simulink model "AUVenv"  (R2025b)
settings: Solver=FixedStepAuto  StartTime=0.0  StopTime=Inf  FixedStep=0.01  RelTol=1e-3
PostLoadFcn:
  | set_param(gcs,'Zoomfactor','fit to view')
undefined symbols (not defined in the file): AUV, fractalcoef, Sim3dSensor, Simple, T200, thrust_pwms, thruster_pose, XYZ
libraries: sim3dlib x7, robotcorelib x5, AUVLib x4, aerolib6dof2 x2, sim3dcameralib x2, matrix_library x1, mspsensorlib x1, aerolibutil x1
(part 1 of 2)
settings Model: Creator=abshanka  LastModifiedBy=ubuntu
settings SolverCC: ZeroCrossAlgorithm=Adaptive
settings DebuggingCC: ReadBeforeWriteMsg=DisableAll  WriteAfterWriteMsg=DisableAll  WriteAfterReadMsg=DisableAll  IgnoredZcDiagnostic=none  MultiTaskDSMMsg=none
settings ModelReferenceCC: UpdateModelReferenceTargets=IfOutOfDate
settings SFSimCC: SFSimEcho=off

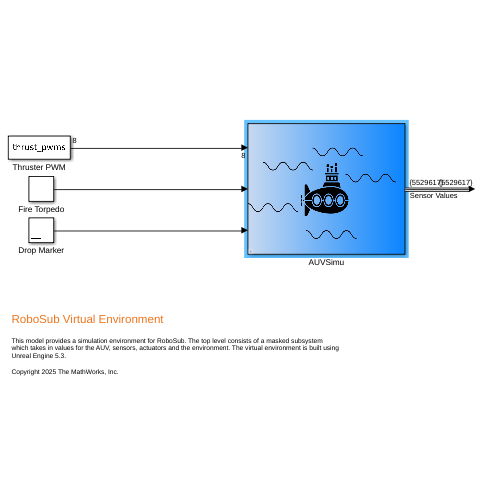
[thumbnail: Simulink's stored preview of the top-level diagram]
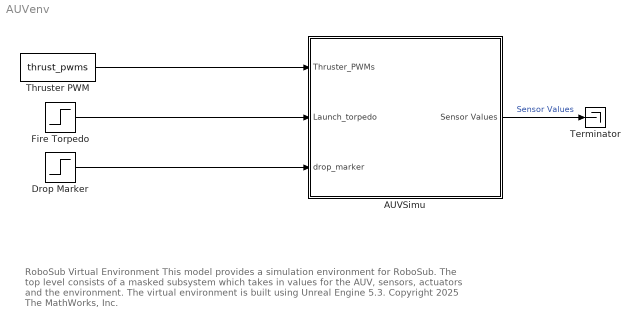
== system AUVenv ==
  note: RoboSub Virtual Environment
      |
      | This model provides a simulation environment for RoboSub. The top level consists of a masked subsystem which takes in values for the AUV, sensors, actuators and the environment. The virtual environment is built using Unreal Engine 5.3.
      |
      | Copyright 2025 The MathWorks, Inc.
  AUVSimu : Subsystem  mask(RoboSub){SourceFile=/home/ubuntu/sonia_control/src/virtual-robosub/fbx files/AUV2.stl, AUV_cob=[0.0026; -0.0004; -0.0911], AUV_height=AUV.Body.hulldiameter, AUV_vol=0.0315, AUV_inertia=AUV.Body.Inertia, AUV_mass=30, AUV_pos=[-142 -142 -1], AUV_orientation=[0 0 pi/2], thruster_pose=thruster_pose, AUV_Voltage=16V, nThrusters=8, Hy=Simple, lin_coeff=diag([ 30,  22,  220]), quad_coeff=diag([ 650,  320,  680]), ang_coeff=diag([ 10, 80,  82]), CMK=AUV.Coeff.CMM, CMM=AUV.Coeff.CMN, CMN=AUV.Coeff.CMK, CZ=AUV.Coeff.CZ, CY=AUV.Coeff.CY, CX=AUV.Coeff.CX, betaR=AUV.IncRange.beta_vec, alphaR=AUV.IncRange.alpha_vec, ang_coeff_c=diag([10, 80, 80]), d_cam_pos=[0 0 -0.26], d_orientation=[0 90 0], SemanticOutportEnabled=off, DepthOutportEnabled=off, TangentialDistortion=[0, 0], RadialDistortion=[0, 0], ImageSize=[720, 1280], OpticalCenter=[640, 360], FocalLength=[1109, 1109], f_cam_pos=[0.5, 0, 0], f_orientation=[0 0 0], SemanticOutportEnabled_f=off, DepthOutportEnabled_f=off, TangentialDistortion_f=[0, 0], RadialDistortion_f=[0, 0], ImageSize_f=[720, 1280], OpticalCenter_f=[640, 360], FocalLength_f=[1109, 1109], ref_mode=Bottom Tracking, Temperature=25, MagneticFieldNED=XYZ, AccelParamsMeasurementRange=Inf, AccelParamsResolution=0, AccelParamsConstantBias=[ 0, 0, 0 ], AccelParamsAxesMisalignment=[ 100, 0, 0; 0, 100, 0; 0, 0, 100 ], AccelParamsNoiseDensity=[ 0, 0, 0 ], AccelParamsBiasInstability=[ 0, 0, 0 ], AccelParamsBiasInstabilityNumerator=fractalcoef().Numerator, AccelParamsBiasInstabilityDenominator=fractalcoef().Denominator, AccelParamsRandomWalk=[ 0, 0, 0 ], AccelParamsNoiseType=double-sided, AccelParamsTemperatureBias=[ 0, 0, 0 ], AccelParamsTemperatureScaleFactor=[ 0, 0, 0 ], GyroParamsMeasurementRange=Inf, GyroParamsResolution=0, GyroParamsConstantBias=[ 0, 0, 0 ], GyroParamsAxesMisalignment=[ 100, 0, 0; 0, 100, 0; 0, 0, 100 ], GyroParamsAccelerationBias=[ 0, 0, 0 ], GyroParamsNoiseDensity=[ 0, 0, 0 ], GyroParamsBiasInstability=[ 0, 0, 0 ], GyroParamsBiasInstabilityNumerator=fractalcoef().Numerator, GyroParamsBiasInstabilityDenominator=fractalcoef().Denominator, GyroParamsRandomWalk=[ 0, 0, 0 ], GyroParamsNoiseType=double-sided, GyroParamsTemperatureBias=[ 0, 0, 0 ], GyroParamsTemperatureScaleFactor=[ 0, 0, 0 ], MagParamsMeasurementRange=Inf, MagParamsResolution=0, MagParamsConstantBias=[ 0, 0, 0 ], MagParamsAxesMisalignment=[ 100, 0, 0; 0, 100, 0; 0, 0, 100 ], MagParamsNoiseDensity=[ 0, 0, 0 ], MagParamsBiasInstability=[ 0, 0, 0 ], MagParamsBiasInstabilityNumerator=fractalcoef().Numerator, MagParamsBiasInstabilityDenominator=fractalcoef().Denominator, MagParamsRandomWalk=[ 0, 0, 0 ], MagParamsNoiseType=double-sided, MagParamsTemperatureBias=[ 0, 0, 0 ], MagParamsTemperatureScaleFactor=[ 0, 0, 0 ], torp_pos=[0.4 0.2 0.1], marker_pos=[-0.01 0 0.02], waterDensity=1000, gravity=9.79624, w_current=None, waterCurrent=[0 0 0], causticsVisibility=off}
      mask prompts: SourceFile "Path to AUV model"; AUV_cob "CoB (relative to CoM) (m)"; AUV_height "Height (or diameter) of AUV (m)"; AUV_vol "Volume of AUV (m^3)"; AUV_inertia "Inerita matrix of AUV"; AUV_mass "Mass of AUV (kg)"; AUV_pos "Inital Position [x,y,z] (m)"; AUV_orientation "Inital Euler Orientation [roll, pith, yaw] (rad)"; thruster_pose "Thruster Pose (nx6 matrix) (m,rad)"; AUV_Voltage "AUV Battery Voltage"; nThrusters "Number of thrusters"; Hy "Choose Hydrodynamics Simulation"; lin_coeff "Linear drag coefficient"; quad_coeff "Quadratic drag coefficient"; ang_coeff "Angular Damping coefficient"; CMK "Rolling moment coeff"; CMM "Pitching moment coeff"; CMN "Yawing moment coeff"; CZ "Normal force coeff (CZ)"; CY "Side force coeff (CY)"; CX "Axial force coeff (CX)"; betaR "Beta Range"; alphaR "Alpha Range"; ang_coeff_c "Angular Damping coefficient"; d_cam_pos "Position (relative to CoM) (m)"; d_orientation "Orientation (deg)"; SemanticOutportEnabled "shared_sim3dblks:sim3dblkCameraPinHole:blkPrm_SemanticOutportEnabled"; DepthOutportEnabled "shared_sim3dblks:sim3dblkCameraPinHole:blkPrm_DepthOutportEnabled"; TangentialDistortion "shared_sim3dblks:sim3dblkCameraPinHole:blkPrm_TangentialDistortion"; RadialDistortion "shared_sim3dblks:sim3dblkCameraPinHole:blkPrm_RadialDistortion"; ImageSize "shared_sim3dblks:sim3dblkCameraPinHole:blkPrm_ImageSize"; OpticalCenter "shared_sim3dblks:sim3dblkCameraPinHole:blkPrm_OpticalCenter"; FocalLength "shared_sim3dblks:sim3dblkCameraPinHole:blkPrm_FocalLength"; f_cam_pos "Position (relative to CoM) (m)"; f_orientation "Orientation (deg)"; SemanticOutportEnabled_f "shared_sim3dblks:sim3dblkCameraPinHole:blkPrm_SemanticOutportEnabled"; DepthOutportEnabled_f "shared_sim3dblks:sim3dblkCameraPinHole:blkPrm_DepthOutportEnabled"; TangentialDistortion_f "shared_sim3dblks:sim3dblkCameraPinHole:blkPrm_TangentialDistortion"; RadialDistortion_f "shared_sim3dblks:sim3dblkCameraPinHole:blkPrm_RadialDistortion"; ImageSize_f "shared_sim3dblks:sim3dblkCameraPinHole:blkPrm_ImageSize"; OpticalCenter_f "shared_sim3dblks:sim3dblkCameraPinHole:blkPrm_OpticalCenter"; FocalLength_f "shared_sim3dblks:sim3dblkCameraPinHole:blkPrm_FocalLength"; ref_mode "Reference mode"; Temperature "Temperature (°C):"; MagneticFieldNED "Magnetic field (NED):"; AccelParamsMeasurementRange "Maximum readings (m/s²):"; AccelParamsResolution "Resolution ((m/s²)/LSB):"; AccelParamsConstantBias "Constant offset bias (m/s²):"; AccelParamsAxesMisalignment "Axes skew (%):"; AccelParamsNoiseDensity "Velocity random walk ((m/s²)/√Hz):"; AccelParamsBiasInstability "Bias instability (m/s²):"; AccelParamsBiasInstabilityNumerator "Bias instability filter numerator coefficients:"; AccelParamsBiasInstabilityDenominator "Bias instability filter denominator coefficients:"; AccelParamsRandomWalk "Acceleration random walk ((m/s²)*√Hz):"; AccelParamsNoiseType "Noise type:"; AccelParamsTemperatureBias "Bias from temperature ((m/s²)/°C):"; AccelParamsTemperatureScaleFactor "Temperature scale factor (%/°C):"; GyroParamsMeasurementRange "Maximum readings (rad/s):"; GyroParamsResolution "Resolution ((rad/s)/LSB):"; GyroParamsConstantBias "Constant offset bias (rad/s):"; GyroParamsAxesMisalignment "Axes skew (%):"; GyroParamsAccelerationBias "Bias from acceleration ((rad/s)/(m/s²)):"; GyroParamsNoiseDensity "Angle random walk ((rad/s)/√Hz):"; GyroParamsBiasInstability "Bias instability (rad/s):"; GyroParamsBiasInstabilityNumerator "Bias instability filter numerator coefficients:"; GyroParamsBiasInstabilityDenominator "Bias instability filter denominator coefficients:"; GyroParamsRandomWalk "Rate random walk ((rad/s)*√Hz):"; GyroParamsNoiseType "Noise type:"; GyroParamsTemperatureBias "Bias from temperature ((rad/s)/°C):"; GyroParamsTemperatureScaleFactor "Temperature scale factor (%/°C):"; MagParamsMeasurementRange "Maximum readings (µT):"; MagParamsResolution "Resolution ((µT)/LSB):"; MagParamsConstantBias "Constant offset bias (µT):"; MagParamsAxesMisalignment "Axes skew (%):"; MagParamsNoiseDensity "White Noise PSD ((µT)/√Hz):"; MagParamsBiasInstability "Bias instability (µT):"; MagParamsBiasInstabilityNumerator "Bias instability filter numerator coefficients:"; MagParamsBiasInstabilityDenominator "Bias instability filter denominator coefficients:"; MagParamsRandomWalk "Random walk ((µT)*√Hz):"; MagParamsNoiseType "Noise type:"; MagParamsTemperatureBias "Bias from temperature ((µT)/°C):"; MagParamsTemperatureScaleFactor "Temperature scale factor (%/°C):"; torp_pos "Torpedo position (m)"; marker_pos "marker_pos (m)"; waterDensity "Water Density (kg/m^3)"; gravity "Acceleration due to Gravity (m/sec^2)"; w_current "Water current"; waterCurrent "Enter current speed in x and y (z=0) (m/s)"; causticsVisibility "Enable Water Caustics"
      mask help:
      | The mask takes in necessary information required to simulate the AUV in a pool. It is divided into 4 sections - AUV Parameters, Sensors, Actuators and Environment.
      | The AUV Parameters section contains all the data related to the AUV body such as mass, inertia, volume, etc. It also takes in the hydrodynamic coefficients (based on the chosen complexity).
      | The Sensors section takes in data related to the sensors such as mounting location and any sensor parameters (for ex: camera - focal lenght, resolution, distortions, etc.)
      | The Actuators sections takes in the mounting location for 2 actuators present in the simulator - torpedo and marker.
      | The Environment section has some parameters related of the environment such as water density, gravity and water currents.
      mask TypeOptions SourceFile: Visualization/AUV mesh/SourceFile
      mask TypeOptions Hy: AUV Dynamics/Environmental Forces and Moments/Hy
      mask TypeOptions lin_coeff: AUV Dynamics/Environmental Forces and Moments/lin_coeff
      mask TypeOptions quad_coeff: AUV Dynamics/Environmental Forces and Moments/quad_coeff
      mask TypeOptions ang_coeff: AUV Dynamics/Environmental Forces and Moments/ang_coeff
      mask TypeOptions CMK: AUV Dynamics/Environmental Forces and Moments/CMK
      mask TypeOptions CMM: AUV Dynamics/Environmental Forces and Moments/CMM
      mask TypeOptions CMN: AUV Dynamics/Environmental Forces and Moments/CMN
      mask TypeOptions CZ: AUV Dynamics/Environmental Forces and Moments/CZ
      mask TypeOptions CY: AUV Dynamics/Environmental Forces and Moments/CY
      mask TypeOptions CX: AUV Dynamics/Environmental Forces and Moments/CX
      mask TypeOptions betaR: AUV Dynamics/Environmental Forces and Moments/betaR
      mask TypeOptions alphaR: AUV Dynamics/Environmental Forces and Moments/alphaR
      mask TypeOptions ang_coeff_c: AUV Dynamics/Environmental Forces and Moments/ang_coeff_c
      mask TypeOptions SemanticOutportEnabled: Sensors/downward_camera/SemanticOutportEnabled
      mask TypeOptions DepthOutportEnabled: Sensors/downward_camera/DepthOutportEnabled
      mask TypeOptions TangentialDistortion: Sensors/downward_camera/TangentialDistortion
      mask TypeOptions RadialDistortion: Sensors/downward_camera/RadialDistortion
      mask TypeOptions ImageSize: Sensors/downward_camera/ImageSize
      mask TypeOptions OpticalCenter: Sensors/downward_camera/OpticalCenter
      mask TypeOptions FocalLength: Sensors/downward_camera/FocalLength
      mask TypeOptions SemanticOutportEnabled_f: Sensors/forward_camera/SemanticOutportEnabled
      mask TypeOptions DepthOutportEnabled_f: Sensors/forward_camera/DepthOutportEnabled
      mask TypeOptions TangentialDistortion_f: Sensors/forward_camera/TangentialDistortion
      mask TypeOptions RadialDistortion_f: Sensors/forward_camera/RadialDistortion
      mask TypeOptions ImageSize_f: Sensors/forward_camera/ImageSize
      mask TypeOptions OpticalCenter_f: Sensors/forward_camera/OpticalCenter
      mask TypeOptions FocalLength_f: Sensors/forward_camera/FocalLength
      mask TypeOptions Temperature: Sensors/IMU Subsystem/IMU/Temperature
      mask TypeOptions MagneticFieldNED: Sensors/IMU Subsystem/IMU/MagneticFieldNED
      mask TypeOptions AccelParamsMeasurementRange: Sensors/IMU Subsystem/IMU/AccelParamsMeasurementRange
      mask TypeOptions AccelParamsResolution: Sensors/IMU Subsystem/IMU/AccelParamsResolution
      mask TypeOptions AccelParamsConstantBias: Sensors/IMU Subsystem/IMU/AccelParamsConstantBias
      mask TypeOptions AccelParamsAxesMisalignment: Sensors/IMU Subsystem/IMU/AccelParamsAxesMisalignment
      mask TypeOptions AccelParamsNoiseDensity: Sensors/IMU Subsystem/IMU/AccelParamsNoiseDensity
      mask TypeOptions AccelParamsBiasInstability: Sensors/IMU Subsystem/IMU/AccelParamsBiasInstability
      mask TypeOptions AccelParamsBiasInstabilityNumerator: Sensors/IMU Subsystem/IMU/AccelParamsBiasInstabilityNumerator
      mask TypeOptions AccelParamsBiasInstabilityDenominator: Sensors/IMU Subsystem/IMU/AccelParamsBiasInstabilityDenominator
      mask TypeOptions AccelParamsRandomWalk: Sensors/IMU Subsystem/IMU/AccelParamsRandomWalk
      mask TypeOptions AccelParamsNoiseType: Sensors/IMU Subsystem/IMU/AccelParamsNoiseType
      mask TypeOptions AccelParamsTemperatureBias: Sensors/IMU Subsystem/IMU/AccelParamsTemperatureBias
      mask TypeOptions AccelParamsTemperatureScaleFactor: Sensors/IMU Subsystem/IMU/AccelParamsTemperatureScaleFactor
      mask TypeOptions GyroParamsMeasurementRange: Sensors/IMU Subsystem/IMU/GyroParamsMeasurementRange
      mask TypeOptions GyroParamsResolution: Sensors/IMU Subsystem/IMU/GyroParamsResolution
      mask TypeOptions GyroParamsConstantBias: Sensors/IMU Subsystem/IMU/GyroParamsConstantBias
      mask TypeOptions GyroParamsAxesMisalignment: Sensors/IMU Subsystem/IMU/GyroParamsAxesMisalignment
      mask TypeOptions GyroParamsAccelerationBias: Sensors/IMU Subsystem/IMU/GyroParamsAccelerationBias
      mask TypeOptions GyroParamsNoiseDensity: Sensors/IMU Subsystem/IMU/GyroParamsNoiseDensity
      mask TypeOptions GyroParamsBiasInstability: Sensors/IMU Subsystem/IMU/GyroParamsBiasInstability
      mask TypeOptions GyroParamsBiasInstabilityNumerator: Sensors/IMU Subsystem/IMU/GyroParamsBiasInstabilityNumerator
      mask TypeOptions GyroParamsBiasInstabilityDenominator: Sensors/IMU Subsystem/IMU/GyroParamsBiasInstabilityDenominator
      mask TypeOptions GyroParamsRandomWalk: Sensors/IMU Subsystem/IMU/GyroParamsRandomWalk
      mask TypeOptions GyroParamsNoiseType: Sensors/IMU Subsystem/IMU/GyroParamsNoiseType
      mask TypeOptions GyroParamsTemperatureBias: Sensors/IMU Subsystem/IMU/GyroParamsTemperatureBias
      mask TypeOptions GyroParamsTemperatureScaleFactor: Sensors/IMU Subsystem/IMU/GyroParamsTemperatureScaleFactor
      mask TypeOptions MagParamsMeasurementRange: Sensors/IMU Subsystem/IMU/MagParamsMeasurementRange
      mask TypeOptions MagParamsResolution: Sensors/IMU Subsystem/IMU/MagParamsResolution
      mask TypeOptions MagParamsConstantBias: Sensors/IMU Subsystem/IMU/MagParamsConstantBias
      mask TypeOptions MagParamsAxesMisalignment: Sensors/IMU Subsystem/IMU/MagParamsAxesMisalignment
      mask TypeOptions MagParamsNoiseDensity: Sensors/IMU Subsystem/IMU/MagParamsNoiseDensity
      mask TypeOptions MagParamsBiasInstability: Sensors/IMU Subsystem/IMU/MagParamsBiasInstability
      mask TypeOptions MagParamsBiasInstabilityNumerator: Sensors/IMU Subsystem/IMU/MagParamsBiasInstabilityNumerator
      mask TypeOptions MagParamsBiasInstabilityDenominator: Sensors/IMU Subsystem/IMU/MagParamsBiasInstabilityDenominator
      mask TypeOptions MagParamsRandomWalk: Sensors/IMU Subsystem/IMU/MagParamsRandomWalk
      mask TypeOptions MagParamsNoiseType: Sensors/IMU Subsystem/IMU/MagParamsNoiseType
      mask TypeOptions MagParamsTemperatureBias: Sensors/IMU Subsystem/IMU/MagParamsTemperatureBias
      mask TypeOptions MagParamsTemperatureScaleFactor: Sensors/IMU Subsystem/IMU/MagParamsTemperatureScaleFactor
      mask DialogControl Container3 Prompt: AUV Parameters
      mask DialogControl Container4 Prompt: General
      mask DialogControl Container5 Prompt: Hydrodynamics
      mask DialogControl Container6 Prompt: Simple hydrodynamics coefficients
      mask DialogControl Container7 Prompt: Complex hydrodynamics coefficients
      mask DialogControl Container8 Prompt: Sensors
      mask DialogControl Container10 Prompt: Downward Camera
      mask DialogControl SemanticOutportEnabled Prompt: Output semantic segmentation
      mask DialogControl DepthOutportEnabled Prompt: Output depth
      mask DialogControl TangentialDistortion Prompt: Tangential distortion coefficients:
      mask DialogControl RadialDistortion Prompt: Radial distortion coefficients:
      mask DialogControl ImageSize Prompt: Image size (pixels):
      mask DialogControl OpticalCenter Prompt: Optical center (pixels):
      mask DialogControl FocalLength Prompt: Focal length (pixels):
      mask DialogControl Container9 Prompt: Forward Camera
      mask DialogControl SemanticOutportEnabled_f Prompt: Output semantic segmentation
      mask DialogControl DepthOutportEnabled_f Prompt: Output depth
      mask DialogControl TangentialDistortion_f Prompt: Tangential distortion coefficients:
      mask DialogControl RadialDistortion_f Prompt: Radial distortion coefficients:
      mask DialogControl ImageSize_f Prompt: Image size (pixels):
      mask DialogControl OpticalCenter_f Prompt: Optical center (pixels):
      mask DialogControl FocalLength_f Prompt: Focal length (pixels):
      mask DialogControl Container11 Prompt: DVL
      mask DialogControl Container12 Prompt: IMU
      mask DialogControl Container16 Prompt: Accelerometer
      mask DialogControl Container17 Prompt: Gyroscope
      mask DialogControl Container18 Prompt: Magnetometer
      mask DialogControl Container13 Prompt: Actuators
      mask DialogControl Container14 Prompt: Environment
      mask Display: image('submarine.png');
  Drop Marker : Step  SampleTime=0
  Fire Torpedo : Step  SampleTime=0
  Terminator : Terminator
  Thruster PWM : Constant  Value=thrust_pwms  SampleTime=0.1
  wires:
  Fire Torpedo/1 -> AUVSimu/2(Launch_torpedo)
  Thruster PWM/1 -> AUVSimu/1(Thruster_PWMs)
  Drop Marker/1 -> AUVSimu/3(drop_marker)
  AUVSimu/1(Sensor Values) -> Terminator/1  "Sensor Values"

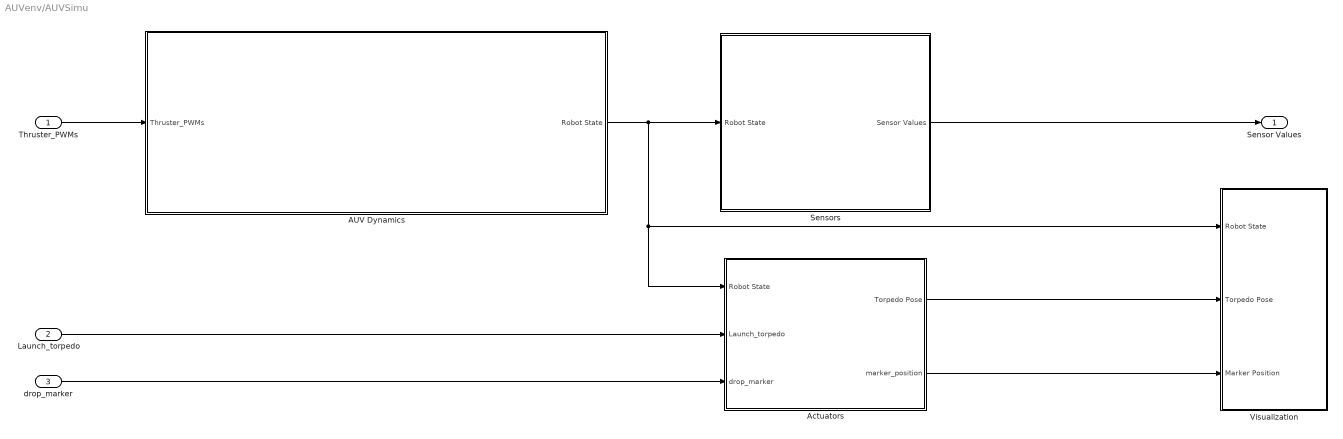
== system AUVenv/AUVSimu ==
  Thruster_PWMs : Inport
  Launch_torpedo : Inport  Port=2
  drop_marker : Inport  Port=3
  AUV Dynamics : Subsystem
  Actuators : Subsystem
  Sensors : Subsystem
  Visualization : Subsystem
  Sensor Values : Outport
  wires:
  Thruster_PWMs/1 -> AUV Dynamics/1(Thruster_PWMs)
  Sensors/1(Sensor Values) -> Sensor Values/1
  AUV Dynamics/1(Robot State) -> Sensors/1(Robot State), Actuators/1(Robot State), Visualization/1(Robot State)
  Launch_torpedo/1 -> Actuators/2(Launch_torpedo)
  drop_marker/1 -> Actuators/3(drop_marker)
  Actuators/1(Torpedo Pose) -> Visualization/2(Torpedo Pose)
  Actuators/2(marker_position) -> Visualization/3(Marker Position)

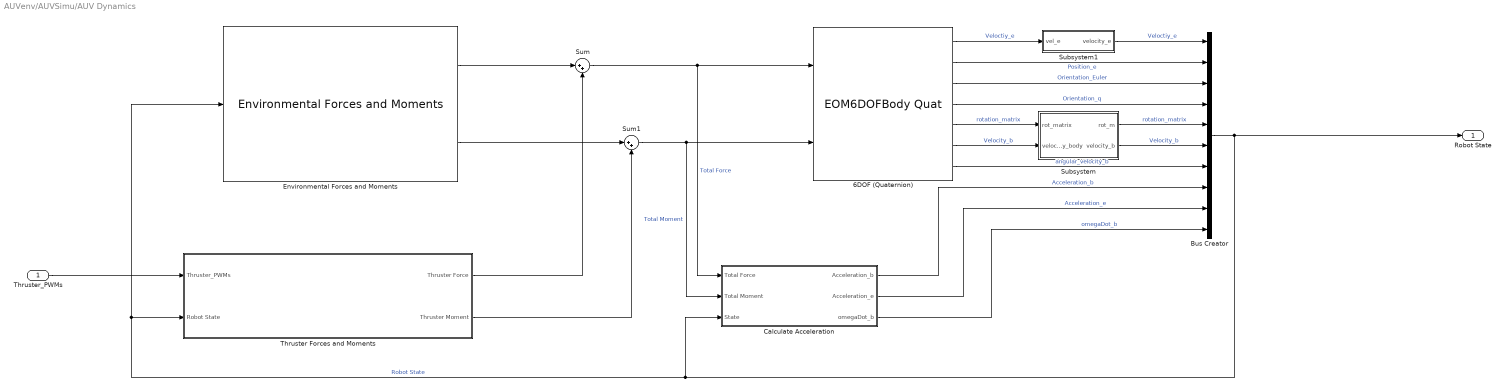
== system AUVenv/AUVSimu/AUV Dynamics ==
  Thruster_PWMs : Inport
  6DOF (Quaternion) : EOM6DOFBodyQuat  xme_0=AUV_pos  eul_0=AUV_orientation  mass_0=AUV_mass  inertia=AUV_inertia
  Bus Creator : BusCreator  Inputs=10
  Calculate Acceleration : Subsystem
  Environmental Forces and Moments : AUVLib/Environmental Forces and Moments  V=AUV_vol  h=AUV_height  mass=AUV_mass  CoB=AUV_cob  Hy=Simple  ang_coeff=ang_coeff  quad_coeff=quad_coeff  lin_coeff=lin_coeff  ang_coeff_c=ang_coeff_c  alphaR=alphaR  betaR=betaR  CX=CX  CY=CY  CZ=CZ  CMK=CMK  CMM=CMM  CMN=CMN  inputAxes=Body  cbar=1  b=1  S=1
  Subsystem : Subsystem
  Subsystem1 : Subsystem
  Sum : Sum  Inputs=|++
  Sum1 : Sum  Inputs=|++
  Thruster Forces and Moments : Subsystem
  Robot State : Outport
  wires:
  6DOF (Quaternion)/3 -> Bus Creator/3  "Orientation_Euler"
  Thruster Forces and Moments/1(Thruster Force) -> Sum/2
  Sum1/1 -> 6DOF (Quaternion)/2, Calculate Acceleration/2(Total Moment)  "Total Moment"
  Thruster Forces and Moments/2(Thruster Moment) -> Sum1/2
  Calculate Acceleration/3(omegaDot_b) -> Bus Creator/10  "omegaDot_b"
  6DOF (Quaternion)/7 -> Bus Creator/7  "angular_velocity_b"
  Sum/1 -> 6DOF (Quaternion)/1, Calculate Acceleration/1(Total Force)  "Total Force"
  Calculate Acceleration/2(Acceleration_e) -> Bus Creator/9  "Acceleration_e"
  6DOF (Quaternion)/1 -> Subsystem1/1(vel_e)  "Veloctiy_e"
  Thruster_PWMs/1 -> Thruster Forces and Moments/1(Thruster_PWMs)
  Calculate Acceleration/1(Acceleration_b) -> Bus Creator/8  "Acceleration_b"
  6DOF (Quaternion)/4 -> Bus Creator/4  "Orientation_q"
  Bus Creator/1 -> Robot State/1, Calculate Acceleration/3(State), Thruster Forces and Moments/2(Robot State), Environmental Forces and Moments/1  "Robot State"
  6DOF (Quaternion)/2 -> Bus Creator/2  "Position_e"
  6DOF (Quaternion)/5 -> Subsystem/1(rot_matrix)  "rotation_matrix"
  6DOF (Quaternion)/6 -> Subsystem/2(velocity_body)  "Velocity_b"
  Subsystem/2(velocity_b) -> Bus Creator/6  "Velocity_b"
  Subsystem/1(rot_m) -> Bus Creator/5  "rotation_matrix"
  Subsystem1/1(velocity_e) -> Bus Creator/1  "Veloctiy_e"
  Environmental Forces and Moments/2 -> Sum1/1
  Environmental Forces and Moments/1 -> Sum/1

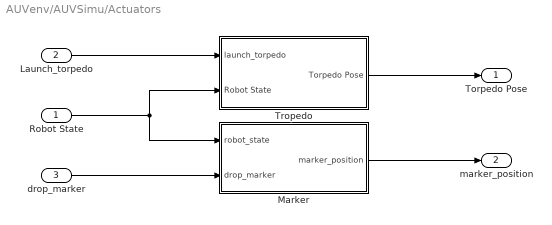
== system AUVenv/AUVSimu/Actuators ==
  Robot State : Inport
  Launch_torpedo : Inport  Port=2
  drop_marker : Inport  Port=3
  Marker : Subsystem
  Tropedo : Subsystem
  Torpedo Pose : Outport
  marker_position : Outport  Port=2
  wires:
  Launch_torpedo/1 -> Tropedo/1(launch_torpedo)
  drop_marker/1 -> Marker/2(drop_marker)
  Robot State/1 -> Marker/1(robot_state), Tropedo/2(Robot State)
  Tropedo/1(Torpedo Pose) -> Torpedo Pose/1
  Marker/1(marker_position) -> marker_position/1

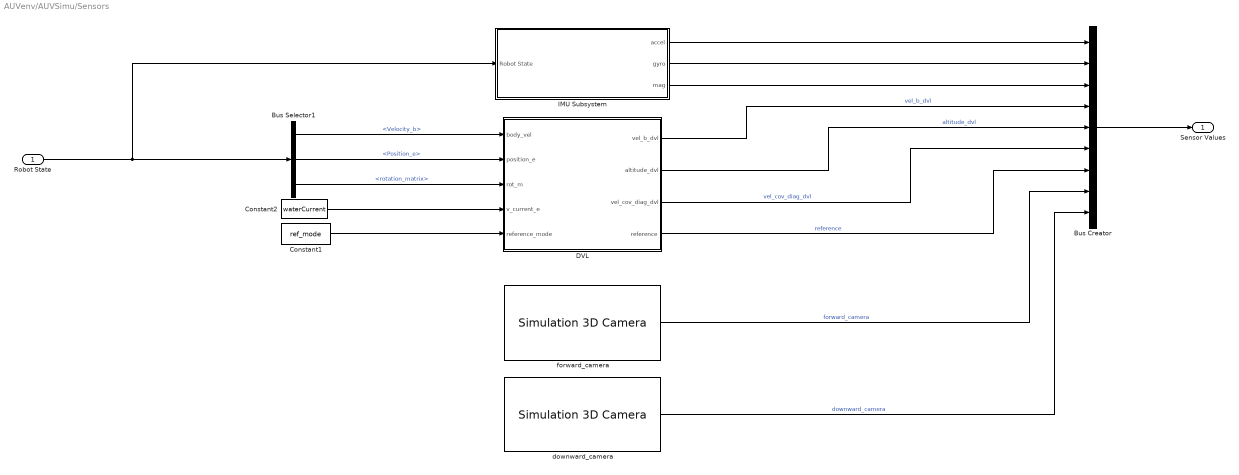
== system AUVenv/AUVSimu/Sensors ==
  Robot State : Inport
  Bus Creator : BusCreator  Inputs=9
  Bus Selector1 : BusSelector  OutputSignals=Velocity_b,Position_e,rotation_matrix
  Constant1 : Constant  Value=ref_mode  OutDataTypeStr=uint8
  Constant2 : Constant  Value=waterCurrent
  DVL : MATLAB Function  TreatAsAtomicUnit=on
  IMU Subsystem : Subsystem
  downward_camera : sim3dcameralib/Simulation 3D Camera  Priority=1  sensorTag=Sim3dSensor�  sensorId=2  sensorName=Sim3dSensor�  vehTagList={'AUVframe';'AUVmesh';'Scene Origin';'marker';'torpedo'}  vehTag=AUVmesh  CoordinateSystem=ISO8855  mountLoc=Origin  offsetFlag=on  tmountOffset=d_cam_pos  extTmount=off  rmountOffset=d_orientation  extRmount=off  FocalLength=FocalLength  OpticalCenter=OpticalCenter  ImageSize=ImageSize  RadialDistortion=RadialDistortion  TangentialDistortion=TangentialDistortion  SensorSkew=0  VisualizeFieldOfView=off  FieldOfViewRange=61  DepthOutportEnabled=off  SemanticOutportEnabled=off  TransformOutportEnabled=off  SampleTime=-1  mountPoint=[0 0 -0.26]  mountOrientation=[0 90 0]  aMode=3  ID=2
      settings: LibrarySourceBlock=drivingsim3d/Simulation 3D Camera
  forward_camera : sim3dcameralib/Simulation 3D Camera  Priority=1  sensorTag=Sim3dSensor�  sensorId=1  sensorName=Sim3dSensor�  vehTagList={'AUVframe';'AUVmesh';'Scene Origin';'marker';'torpedo'}  vehTag=AUVmesh  CoordinateSystem=ISO8855  mountLoc=Origin  offsetFlag=on  tmountOffset=f_cam_pos  extTmount=off  rmountOffset=f_orientation  extRmount=off  FocalLength=FocalLength_f  OpticalCenter=OpticalCenter_f  ImageSize=ImageSize_f  RadialDistortion=RadialDistortion_f  TangentialDistortion=TangentialDistortion_f  SensorSkew=0  VisualizeFieldOfView=off  FieldOfViewRange=61  DepthOutportEnabled=off  SemanticOutportEnabled=off  TransformOutportEnabled=off  SampleTime=-1  mountPoint=[0.5 0 0]  mountOrientation=[0 0 0]  aMode=6  ID=1
      settings: LibrarySourceBlock=robotsim3dlib/Simulation 3D Camera
  Sensor Values : Outport
  wires:
  Robot State/1 -> IMU Subsystem/1(Robot State), Bus Selector1/1
  Bus Selector1/1 -> DVL/1(body_vel)  "<Velocity_b>"
  Bus Selector1/2 -> DVL/2(position_e)  "<Position_e>"
  Bus Selector1/3 -> DVL/3(rot_m)  "<rotation_matrix>"
  Constant2/1 -> DVL/4(v_current_e)
  Constant1/1 -> DVL/5(reference_mode)
  DVL/1(vel_b_dvl) -> Bus Creator/4  "vel_b_dvl"
  DVL/2(altitude_dvl) -> Bus Creator/5  "altitude_dvl"
  DVL/3(vel_cov_diag_dvl) -> Bus Creator/6  "vel_cov_diag_dvl"
  DVL/4(reference) -> Bus Creator/7  "reference"
  Bus Creator/1 -> Sensor Values/1
  forward_camera/1 -> Bus Creator/8  "forward_camera"
  downward_camera/1 -> Bus Creator/9  "downward_camera"
  IMU Subsystem/1(accel) -> Bus Creator/1
  IMU Subsystem/2(gyro) -> Bus Creator/2
  IMU Subsystem/3(mag) -> Bus Creator/3

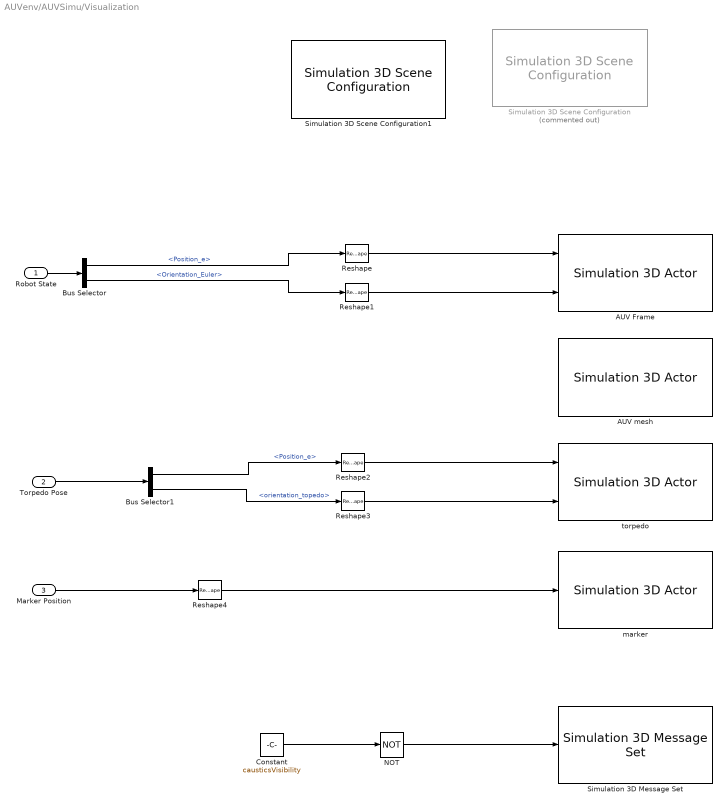
== system AUVenv/AUVSimu/Visualization ==
  Robot State : Inport
  Torpedo Pose : Inport  Port=2
  Marker Position : Inport  Port=3
  AUV Frame : sim3dlib/Simulation 3D Actor  Priority=1  ActorName=AUVframe  ParentName=Scene Origin  Operation=Create at setup  InitScriptText=|  SampleTime=-1  Translation=[0 0 0]  Rotation=[0 0 0]  Scale=[1 1 1]  InputsText=AUVframe.Translation AUVframe.Rotation  aMode=5  ActorTag=AUVframe  ActorType=Sim3dActor  ID=C
      | Actor.CoordinateSystem = 'AERO';
      | Actor.Collisions = false;
  AUV mesh : sim3dlib/Simulation 3D Actor  Priority=1  ActorName=AUVmesh  ParentName=AUVframe  Operation=Create at setup  InitScriptText=|  SampleTime=-1  Translation=[0 0 0]  Rotation=[0 0 0]  Scale=[1 1 1]  aMode=5  ActorTag=AUVmesh  ActorType=Sim3dActor  ID=C
      | Actor.CoordinateSystem = 'AERO';
      | % createShape(Actor, 'Cylinder', [1 0.5 0.5]);
      | Actor.Collisions = false;
  Bus Selector : BusSelector  OutputSignals=Position_e,Orientation_Euler
  Bus Selector1 : BusSelector  OutputSignals=Position_e,orientation_topedo
  Constant : Constant  Value=causticsVisibility  OutDataTypeStr=boolean
  NOT : Logic  Operator=NOT  IconShape=distinctive  AllPortsSameDT=off  OutDataTypeStr=boolean
  Reshape{,1..4} (5 alike) : Reshape  OutputDimensionality=Row vector (2-D)
  Simulation 3D Message Set : sim3dlib/Simulation 3D Message Set  Priority=-1  SigName=causticsVis  Ts=0.01  aMode=0
      settings: LibrarySourceBlock=aerolibsim3d/Simulation 3D Message Set
  Simulation 3D Scene Configuration : sim3dlib/Simulation 3D Scene Configuration  Priority=0  Commented=on  ProjectFormat=Unreal Executable  SceneDesc=Empty scene  ProjectName=/home/ubuntu/simu-sonia/RoboSub_pool_25b/AutoVrtlEnv.exe  ScenePath=/Game/Maps/RoboSub_pool  EnableOpenDRIVE=off  vehTagList={'AUVframe';'AUVmesh';'Custom';'Custom_pool';'Scene Origin';'marker';'torpedo'}  vehTag=Custom_pool  AttachedCameraRelativeTranslation=[0 0 0]  FreeCameraDefaultInitialTranslation=[-6, 0, 2]  AttachedCameraRelativeRotation=[0 0 0]  FreeCameraDefaultInitialRotation=[0, -15, 0]  ViewpointName=Custom_pool  FreeCameraInitialTranslation=[-150 -142 2.5]  ViewpointTranslation=[0 0 0]  FreeCameraInitialRotation=[0 0 0]  ViewpointRotation=[0 0 0]  OpVisEn=off  Ts=.01  EnableWindow=on  EnableRemoteAccess=off  EnableWeather=off  SunAzimuth=90  SunAltitude=40.0  EnableGeospatialSun=off  Latitude=0  Longitude=0  Date=2023-01-01  Time=10:30:00  GeoTimeZone=-5.0  SunDaylightSaving=off  wind=1  clouds=10  EnableVolumetricClouds=off  CloudCoverage=0  CloudAltitude=6  fog=0  rain=0  RaindropsEffect=off  SnowDensity=0  EnableGeospatial=off  TilesetSource=Earth terrain  UseTrueOrigin=off  OriginHeight=200  OriginLatitude=40.744652  OriginLongitude=-73.988864  MapStyle=Aerial  AdditionalAssetIDs=[]  UseAdvancedSunSky=off  SolarTime=11  TimeZone=-5  Day=21  Month=9  Year=2022  UseDaylightSavingTime=on  DSTStartDay=10  DSTStartMonth=3  DSTEndDay=3  DSTEndMonth=11  DSTSwitchHour=2  sensorTag=MainCamera1  sensorId=1  sensorName=MainCamera1  mountLoc=Origin  offsetFlag=off  tmountOffset=[0, 0, 0]  rmountOffset=[0, 0, 0]  HorizontalResolution=1280  VerticalResolution=720  HorizontalFOV=60  mountPoint=[0 0 0]  mountOrientation=[0 0 0]  aMode=5  ID=1  GeoTrigger=Inactive  ViewNameList={'Custom', 'Custom_pool'}  ViewTranslationList={'[-100 -100 1]', '[-150 -142 2.5]'}  ViewRotationList={'[0 0 0]', '[0 0 0]'}
      settings: LibrarySourceBlock=sl3dlib/Simulation 3D/Environment/Simulation 3D Scene Configuration
  Simulation 3D Scene Configuration1 : sim3dlib/Simulation 3D Scene Configuration  Priority=0  ProjectFormat=Default Scenes  SceneDesc=Straight road  ProjectName=/usr/local/MATLAB/R2025b/toolbox/shared/sim3d_projects/automotive_project_linux/UE/LinuxNoEditor/VehicleSimulation.sh  ScenePath=/Game/Maps/RoboSub_pool  EnableOpenDRIVE=off  vehTagList={'AUVframe';'AUVmesh';'Custom';'Custom_pool';'Scene Origin';'marker';'torpedo'}  vehTag=Custom_pool  AttachedCameraRelativeTranslation=[0 0 0]  FreeCameraDefaultInitialTranslation=[-6, 0, 2]  AttachedCameraRelativeRotation=[0 0 0]  FreeCameraDefaultInitialRotation=[0, -15, 0]  ViewpointName=Custom_pool  FreeCameraInitialTranslation=[-150 -142 2.5]  ViewpointTranslation=[0 0 0]  FreeCameraInitialRotation=[0 0 0]  ViewpointRotation=[0 0 0]  OpVisEn=off  Ts=.01  EnableWindow=on  EnableRemoteAccess=off  EnableWeather=off  SunAzimuth=90  SunAltitude=40.0  EnableGeospatialSun=off  Latitude=0  Longitude=0  Date=2023-01-01  Time=10:30:00  GeoTimeZone=-5.0  SunDaylightSaving=off  wind=1  clouds=10  EnableVolumetricClouds=off  CloudCoverage=0  CloudAltitude=6  fog=0  rain=0  RaindropsEffect=off  SnowDensity=0  EnableGeospatial=off  TilesetSource=Earth terrain  UseTrueOrigin=off  OriginHeight=200  OriginLatitude=40.744652  OriginLongitude=-73.988864  MapStyle=Aerial  AdditionalAssetIDs=[]  UseAdvancedSunSky=off  SolarTime=11  TimeZone=-5  Day=21  Month=9  Year=2022  UseDaylightSavingTime=on  DSTStartDay=10  DSTStartMonth=3  DSTEndDay=3  DSTEndMonth=11  DSTSwitchHour=2  sensorTag=MainCamera2  sensorId=2  sensorName=MainCamera2  mountLoc=Origin  offsetFlag=off  tmountOffset=[0, 0, 0]  rmountOffset=[0, 0, 0]  HorizontalResolution=1280  VerticalResolution=720  HorizontalFOV=60  mountPoint=[0 0 0]  mountOrientation=[0 0 0]  aMode=5  ID=2  GeoTrigger=Inactive  ViewNameList={'Custom', 'Custom_pool'}  ViewTranslationList={'[-100 -100 1]', '[-150 -142 2.5]'}  ViewRotationList={'[0 0 0]', '[0 0 0]'}
      settings: LibrarySourceBlock=sl3dlib/Simulation 3D/Environment/Simulation 3D Scene Configuration
  marker : sim3dlib/Simulation 3D Actor  Priority=1  ActorName=marker  ParentName=Scene Origin  Operation=Create at setup  InitScriptText=|  SampleTime=-1  Translation=[0 0 0]  Rotation=[0 0 pi/2]  Scale=[1 1 1]  InputsText=marker.Translation  aMode=5  ActorTag=marker  ActorType=Sim3dActor  ID=C
      | % Reserved keywords:
      | % - Actor : handle to this actor object
      | % - World : handle to the world object
      | 
      | % Examples:
      | 
      | % Create a primitive geometry (optional)
      | % createShape(Actor, 'box', [1 1 1]);
      | 
      | % Initialize values (optional)
      | % Actor.Physics = true;
      | % Actor.Color = [1 0 0];
      | Actor.CoordinateSystem = 'AERO';
      | createShape(Actor, 'sphere', [0.1 0.1 0.1]);
      | Actor.Color = [0 1 0];
  torpedo : sim3dlib/Simulation 3D Actor  Priority=1  ActorName=torpedo  ParentName=SceneOrigin  Operation=Create at setup  InitScriptText=|  SampleTime=-1  Translation=[0 0.27 0]  Rotation=[0 0 pi/2]  Scale=[1 1 1]  InputsText=torpedo.Translation torpedo.Rotation  aMode=5  ActorTag=torpedo  ActorType=Sim3dActor  ID=C
      | % Reserved keywords:
      | % - Actor : handle to this actor object
      | % - World : handle to the world object
      | 
      | % Examples:
      | 
      | % Create a primitive geometry (optional)
      | % createShape(Actor, 'box', [1 1 1]);
      | 
      | % Initialize values (optional)
      | % Actor.Physics = true;
      | % Actor.Color = [1 0 0];
      | Actor.CoordinateSystem = 'AERO';
      | createShape(Actor, 'box', [0.15 0.01 0.01]);
      | Actor.Color = [1 0 0];
  wires:
  Torpedo Pose/1 -> Bus Selector1/1
  Robot State/1 -> Bus Selector/1
  Bus Selector/1 -> Reshape/1  "<Position_e>"
  Bus Selector/2 -> Reshape1/1  "<Orientation_Euler>"
  Reshape/1 -> AUV Frame/1
  Reshape2/1 -> torpedo/1
  Reshape3/1 -> torpedo/2
  Bus Selector1/1 -> Reshape2/1  "<Position_e>"
  Marker Position/1 -> Reshape4/1
  Reshape4/1 -> marker/1
  Reshape1/1 -> AUV Frame/2
  Bus Selector1/2 -> Reshape3/1  "<orientation_topedo>"
  Constant/1 -> NOT/1
  NOT/1 -> Simulation 3D Message Set/1

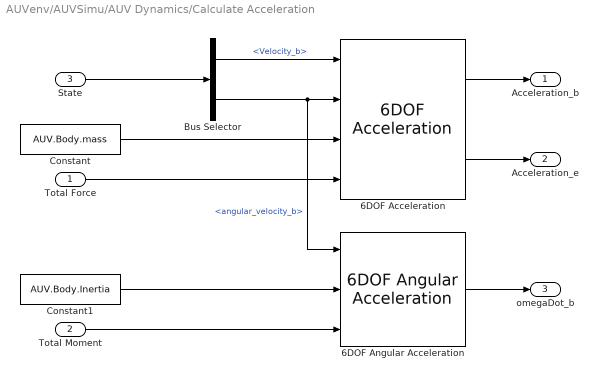
== system AUVenv/AUVSimu/AUV Dynamics/Calculate Acceleration ==
  Total Force : Inport
  Total Moment : Inport  Port=2
  State : Inport  Port=3
  6DOF Acceleration : aerolib6dof2/6DOF Acceleration  units=Metric (MKS)  mtype=Fixed  vre_flag=off
  6DOF Angular Acceleration : aerolib6dof2/6DOF Angular Acceleration  units=Metric (MKS)  mtype=Fixed
  Bus Selector : BusSelector  OutputSignals=Velocity_b,angular_velocity_b
  Constant : Constant  Value=AUV.Body.mass
  Constant1 : Constant  Value=AUV.Body.Inertia
  Acceleration_b : Outport
  Acceleration_e : Outport  Port=2
  omegaDot_b : Outport  Port=3
  wires:
  Constant/1 -> 6DOF Acceleration/3
  Bus Selector/2 -> 6DOF Angular Acceleration/1, 6DOF Acceleration/2  "<angular_velocity_b>"
  Total Moment/1 -> 6DOF Angular Acceleration/3
  State/1 -> Bus Selector/1
  Total Force/1 -> 6DOF Acceleration/4
  Bus Selector/1 -> 6DOF Acceleration/1  "<Velocity_b>"
  Constant1/1 -> 6DOF Angular Acceleration/2
  6DOF Acceleration/1 -> Acceleration_b/1
  6DOF Angular Acceleration/1 -> omegaDot_b/1
  6DOF Acceleration/2 -> Acceleration_e/1

== system AUVenv/AUVSimu/AUV Dynamics/Subsystem ==
  rot_matrix : Inport
  velocity_body : Inport  Port=2
  Matrix Multiply : Product  Multiplication=Matrix(*)
  Sum : Sum  Inputs=|-+
  currentVelocity_e : Constant  Value=waterCurrent
  rot_m : Outport
  velocity_b : Outport  Port=2
  wires:
  currentVelocity_e/1 -> Matrix Multiply/2
  rot_matrix/1 -> Matrix Multiply/1, rot_m/1
  velocity_body/1 -> Sum/2
  Sum/1 -> velocity_b/1
  Matrix Multiply/1 -> Sum/1

== system AUVenv/AUVSimu/AUV Dynamics/Subsystem1 ==
  vel_e : Inport
  Sum : Sum  Inputs=|++
  currentVelocity : Constant  Value=waterCurrent
  velocity_e : Outport
  wires:
  vel_e/1 -> Sum/1
  Sum/1 -> velocity_e/1
  currentVelocity/1 -> Sum/2

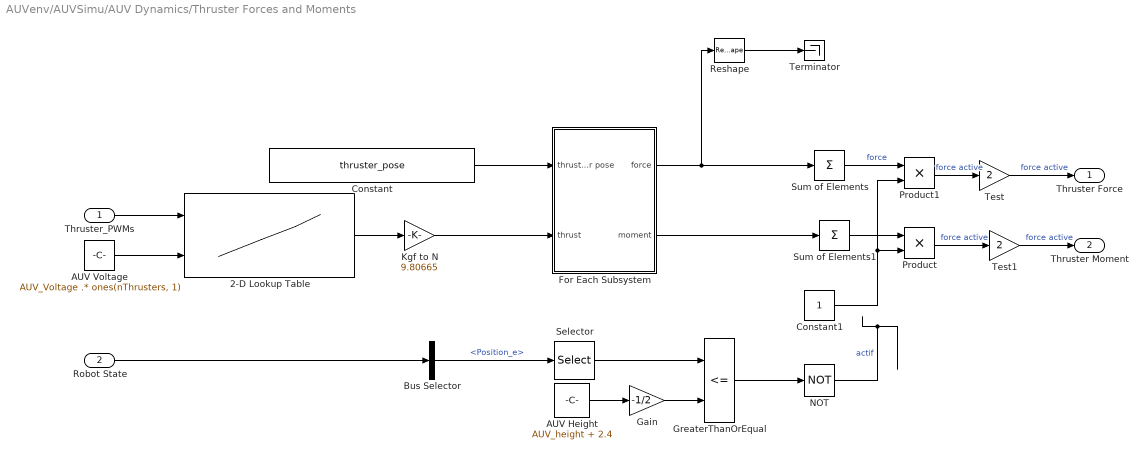
== system AUVenv/AUVSimu/AUV Dynamics/Thruster Forces and Moments ==
  Thruster_PWMs : Inport
  Robot State : Inport  Port=2
  2-D Lookup Table : Lookup_n-D  BreakpointsForDimension1=T200.pwm  BreakpointsForDimension2=T200.voltages  Table=T200.thrust  InternalRulePriority=Speed  RndMeth=Simplest
      settings: InputPortMap=u0,u1
  AUV Height : Constant  Value=AUV_height + 2.4
  AUV Voltage : Constant  Value=AUV_Voltage .* ones(nThrusters, 1)
  Bus Selector : BusSelector  OutputSignals=Position_e
  Constant : Constant  Value=thruster_pose
  Constant1 : Constant
  For Each Subsystem : Subsystem  TreatAsAtomicUnit=on
  Gain : Gain  Gain=-1/2
  GreaterThanOrEqual : RelationalOperator  Operator=<=  OutDataTypeStr=boolean  RndMeth=Simplest  InputSameDT=off
  Kgf to N : Gain  Gain=9.80665
  NOT : Logic  Operator=NOT  IconShape=distinctive  AllPortsSameDT=off  OutDataTypeStr=boolean
  Product : Product
  Product1 : Product
  Reshape : Reshape  OutputDimensionality=Column vector (2-D)
  Selector : Selector  InputPortWidth=3  IndexOptions=Index vector (dialog)  Indices=[3]  OutputSizes=1
  Sum of Elements : Sum  Inputs=+  CollapseMode=Specified dimension
  Sum of Elements1 : Sum  Inputs=+  CollapseMode=Specified dimension
  Terminator : Terminator
  Test : Gain  Gain=2
  Test1 : Gain  Gain=2
  Thruster Force : Outport
  Thruster Moment : Outport  Port=2
  wires:
  Constant/1 -> For Each Subsystem/1(thruster pose)
  For Each Subsystem/2(moment) -> Sum of Elements1/1
  For Each Subsystem/1(force) -> Reshape/1, Sum of Elements/1
  Robot State/1 -> Bus Selector/1
  Bus Selector/1 -> Selector/1  "<Position_e>"
  AUV Height/1 -> Gain/1
  Selector/1 -> GreaterThanOrEqual/1
  Gain/1 -> GreaterThanOrEqual/2
  Sum of Elements/1 -> Product1/1  "force"
  Product1/1 -> Test/1  "force active"
  Sum of Elements1/1 -> Product/1
  Product/1 -> Test1/1  "force active"
  GreaterThanOrEqual/1 -> NOT/1
  NOT/1 -> ?  "actif"
  Thruster_PWMs/1 -> 2-D Lookup Table/1
  2-D Lookup Table/1 -> Kgf to N/1
  AUV Voltage/1 -> 2-D Lookup Table/2
  Kgf to N/1 -> For Each Subsystem/2(thrust)
  Constant1/1 -> Product1/2, Product/2
  Test/1 -> Thruster Force/1  "force active"
  Test1/1 -> Thruster Moment/1  "force active"
  Reshape/1 -> Terminator/1

== system AUVenv/AUVSimu/Actuators/Marker ==
  robot_state : Inport
  drop_marker : Inport  Port=2
  Get Inital state : AUVLib/Get Inital state  SystemSampleTime=-1  VariantActivationTime=update diagram  EmptyChoice=off  PassThrough=off  PassThroughVariantControl=(default)  EmptyChoiceVariantControl=(default)  AllowFlexibleInterface=on  Latency=0  AutoFrameSizeCalculation=off
  Marker Dynamics : Subsystem  TreatAsAtomicUnit=on
  marker_position : Outport
  wires:
  robot_state/1 -> Get Inital state/1
  Get Inital state/1 -> Marker Dynamics/1(Initial_state)
  drop_marker/1 -> Get Inital state/Trigger, Marker Dynamics/Enable
  Marker Dynamics/1(marker_position) -> marker_position/1

== system AUVenv/AUVSimu/Actuators/Tropedo ==
  launch_torpedo : Inport
  Robot State : Inport  Port=2
  Get Inital state : AUVLib/Get Inital state  SystemSampleTime=-1  VariantActivationTime=update diagram  EmptyChoice=off  PassThrough=off  PassThroughVariantControl=(default)  EmptyChoiceVariantControl=(default)  AllowFlexibleInterface=on  Latency=0  AutoFrameSizeCalculation=off
  Torpedo Dynamics : Subsystem  TreatAsAtomicUnit=on
  Torpedo Pose : Outport
  wires:
  Get Inital state/1 -> Torpedo Dynamics/1(Initial_state)
  launch_torpedo/1 -> Get Inital state/Trigger, Torpedo Dynamics/Enable
  Robot State/1 -> Get Inital state/1
  Torpedo Dynamics/1(Torpedo Pose) -> Torpedo Pose/1

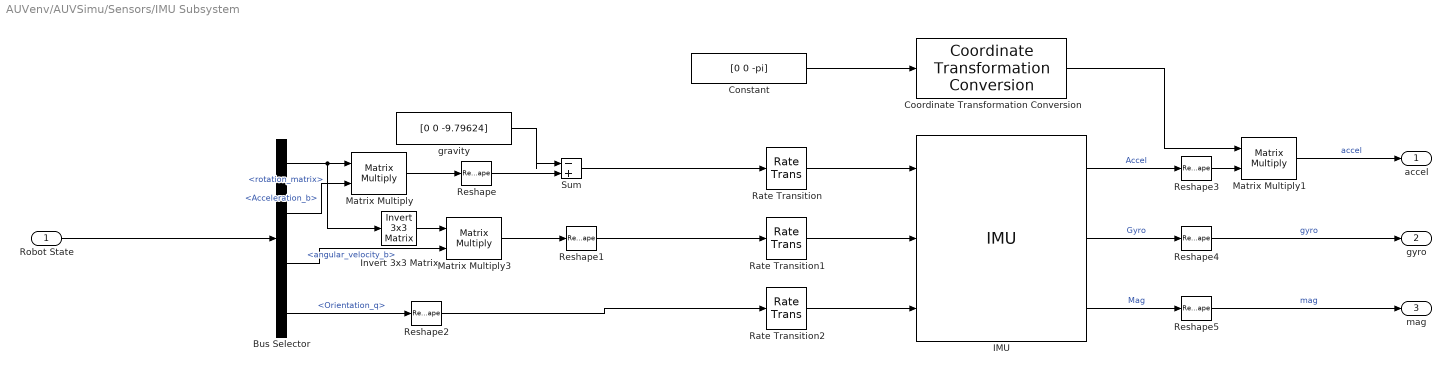
== system AUVenv/AUVSimu/Sensors/IMU Subsystem ==
  Robot State : Inport
  Bus Selector : BusSelector  OutputSignals=rotation_matrix,Acceleration_b,angular_velocity_b,Orientation_q
  Constant : Constant  Value=[0 0 -pi]
  Coordinate Transformation Conversion : robotcorelib/Coordinate Transformation Conversion  InputRepresentation=Euler Angles  InputEulerSequence=ZYX  ShowTrVecInputPort=on  OutputRepresentation=Rotation Matrix  OutputEulerSequence=ZYX  ShowTrVecOutputPort=on  SimulateUsing=Interpreted execution
      settings: LibrarySourceBlock=navlib/Utilities/Coordinate Transformation Conversion
  IMU : mspsensorlib/IMU  DispRefFrame=NED  TemperaturePort=off  Temperature=Temperature  MagneticFieldPort=off  MagneticFieldNED=MagneticFieldNED  MagneticFieldENU=[ -2.4169, 27.5550, 16.0849 ]  SeedDouble=67  SimulateUsing=Interpreted execution  AccelParamsMeasurementRange=AccelParamsMeasurementRange  AccelParamsResolution=AccelParamsResolution  AccelParamsConstantBias=AccelParamsConstantBias  AccelParamsAxesMisalignment=AccelParamsAxesMisalignment  AccelParamsNoiseDensity=AccelParamsNoiseDensity  AccelParamsBiasInstability=AccelParamsBiasInstability  AccelParamsBiasInstabilityNumerator=AccelParamsBiasInstabilityNumerator  AccelParamsBiasInstabilityDenominator=AccelParamsBiasInstabilityDenominator  AccelParamsRandomWalk=AccelParamsRandomWalk  AccelParamsNoiseType=double-sided  AccelParamsTemperatureBias=AccelParamsTemperatureBias  AccelParamsTemperatureScaleFactor=AccelParamsTemperatureScaleFactor  GyroParamsMeasurementRange=GyroParamsMeasurementRange  GyroParamsResolution=GyroParamsResolution  GyroParamsConstantBias=GyroParamsConstantBias  GyroParamsAxesMisalignment=GyroParamsAxesMisalignment  GyroParamsAccelerationBias=GyroParamsAccelerationBias  GyroParamsNoiseDensity=GyroParamsNoiseDensity  GyroParamsBiasInstability=GyroParamsBiasInstability  GyroParamsBiasInstabilityNumerator=GyroParamsBiasInstabilityNumerator  GyroParamsBiasInstabilityDenominator=GyroParamsBiasInstabilityDenominator  GyroParamsRandomWalk=GyroParamsRandomWalk  GyroParamsNoiseType=double-sided  GyroParamsTemperatureBias=GyroParamsTemperatureBias  GyroParamsTemperatureScaleFactor=GyroParamsTemperatureScaleFactor  MagParamsMeasurementRange=MagParamsMeasurementRange  MagParamsResolution=MagParamsResolution  MagParamsConstantBias=MagParamsConstantBias  MagParamsAxesMisalignment=MagParamsAxesMisalignment  MagParamsNoiseDensity=MagParamsNoiseDensity  MagParamsBiasInstability=MagParamsBiasInstability  MagParamsBiasInstabilityNumerator=MagParamsBiasInstabilityNumerator  MagParamsBiasInstabilityDenominator=MagParamsBiasInstabilityDenominator  MagParamsRandomWalk=MagParamsRandomWalk  MagParamsNoiseType=double-sided  MagParamsTemperatureBias=MagParamsTemperatureBias  MagParamsTemperatureScaleFactor=MagParamsTemperatureScaleFactor
  Invert 3x3 Matrix : aerolibutil/Invert  3x3 Matrix
  Matrix Multiply : Product  Multiplication=Matrix(*)
  Matrix Multiply1 : Product  Multiplication=Matrix(*)
  Matrix Multiply3 : Product  Multiplication=Matrix(*)
  Rate Transition : RateTransition
  Rate Transition1 : RateTransition
  Rate Transition2 : RateTransition
  Reshape : Reshape  OutputDimensionality=Row vector (2-D)
  Reshape1 : Reshape  OutputDimensionality=Row vector (2-D)
  Reshape2 : Reshape  OutputDimensionality=Row vector (2-D)
  Reshape3 : Reshape  OutputDimensionality=Column vector (2-D)
  Reshape4 : Reshape  OutputDimensionality=Column vector (2-D)
  Reshape5 : Reshape  OutputDimensionality=Column vector (2-D)
  Sum : Sum  Inputs=|-+
  gravity : Constant  Value=[0 0 -9.79624]
  accel : Outport
  gyro : Outport  Port=2
  mag : Outport  Port=3
  wires:
  Rate Transition1/1 -> IMU/2
  Rate Transition2/1 -> IMU/3
  gravity/1 -> Sum/1
  Reshape/1 -> Sum/2
  Bus Selector/3 -> Matrix Multiply3/2  "<angular_velocity_b>"
  Sum/1 -> Rate Transition/1
  Reshape2/1 -> Rate Transition2/1
  Invert 3x3 Matrix/1 -> Matrix Multiply3/1
  Matrix Multiply1/1 -> accel/1  "accel"
  IMU/2 -> Reshape4/1  "Gyro"
  Matrix Multiply/1 -> Reshape/1
  Matrix Multiply3/1 -> Reshape1/1
  Rate Transition/1 -> IMU/1
  Coordinate Transformation Conversion/1 -> Matrix Multiply1/1
  Bus Selector/2 -> Matrix Multiply/2  "<Acceleration_b>"
  Bus Selector/4 -> Reshape2/1  "<Orientation_q>"
  IMU/1 -> Reshape3/1  "Accel"
  Robot State/1 -> Bus Selector/1
  Constant/1 -> Coordinate Transformation Conversion/1
  Bus Selector/1 -> Invert 3x3 Matrix/1, Matrix Multiply/1  "<rotation_matrix>"
  Reshape3/1 -> Matrix Multiply1/2
  Reshape1/1 -> Rate Transition1/1
  IMU/3 -> Reshape5/1  "Mag"
  Reshape4/1 -> gyro/1  "gyro"
  Reshape5/1 -> mag/1  "mag"

== system AUVenv/AUVSimu/AUV Dynamics/Thruster Forces and Moments/For Each Subsystem ==
  thruster pose : Inport  Partition=on  PartitionDimension=1  PartitionWidth=1  PartitionOffset=0
  thrust : Inport  Port=2  Partition=on  PartitionDimension=1  PartitionWidth=1  PartitionOffset=0
  Calculate Force and Moment : Subsystem
  For Each : ForEach  DisableCoverage=on
  force : Outport  ConcatenationDimension=1
  moment : Outport  Port=2  ConcatenationDimension=1
  wires:
  thruster pose/1 -> Calculate Force and Moment/1(thruster pose)
  Calculate Force and Moment/2(moment) -> moment/1
  Calculate Force and Moment/1(force) -> force/1
  thrust/1 -> Calculate Force and Moment/2(Thrust)

== system AUVenv/AUVSimu/Actuators/Marker/Marker Dynamics ==
  Initial_state : Inport
  drop_marker : EnablePort
  Bus Selector : BusSelector  OutputSignals=Position_e,Veloctiy_e,rotation_matrix
  Constant : Constant  Value=[marker_pos(1) marker_pos(2) -marker_pos(3)]
  MATLAB Function : MATLAB Function  TreatAsAtomicUnit=on
  Scope : Scope
      settings: ActiveDisplayYMinimum=-8.92103223977475  ActiveDisplayYMaximum=3.8325960679282667  DataLoggingVariableName=ScopeData4
  marker_position : Outport
  wires:
  MATLAB Function/1(marker_position) -> Scope/1, marker_position/1
  Initial_state/1 -> Bus Selector/1
  Bus Selector/1 -> MATLAB Function/1(init_pos)  "<Position_e>"
  Bus Selector/2 -> MATLAB Function/2(init_velocity)  "<Veloctiy_e>"
  Bus Selector/3 -> MATLAB Function/3(rot_m)  "<rotation_matrix>"
  Constant/1 -> MATLAB Function/4(marker_loc_b)

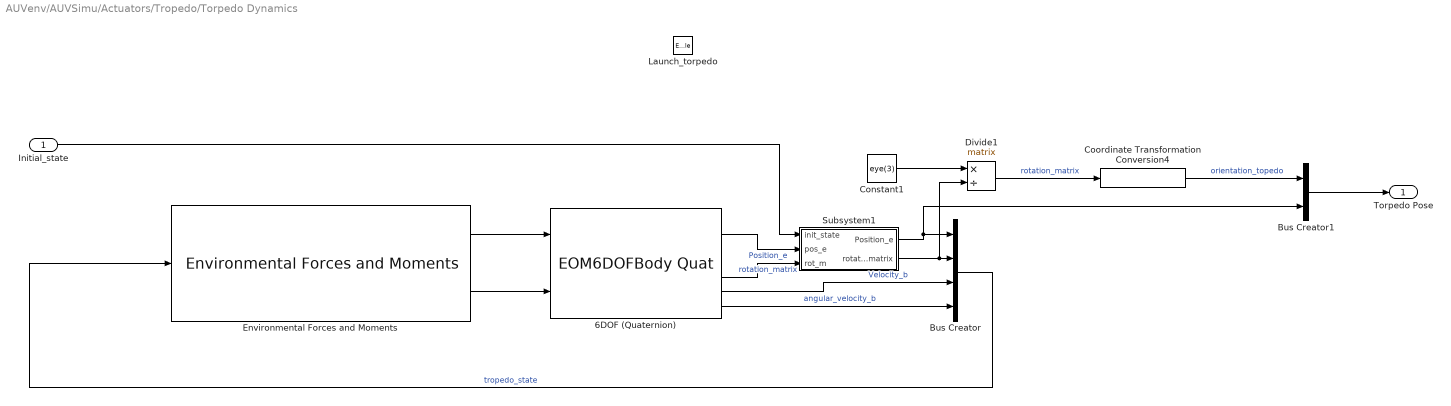
== system AUVenv/AUVSimu/Actuators/Tropedo/Torpedo Dynamics ==
  Initial_state : Inport
  Launch_torpedo : EnablePort
  6DOF (Quaternion) : EOM6DOFBodyQuat  xme_0=torp_pos  Vm_0=[10 0 0]  mass_0=0.02  inertia=[0.02 0 0; 0 0.5 0; 0 0 0.5]
  Bus Creator : BusCreator  Inputs=4
  Bus Creator1 : BusCreator  Inputs=2
  Constant1 : Constant  Value=eye(3)
  Coordinate Transformation Conversion4 : robotcorelib/Coordinate Transformation Conversion  InputRepresentation=Rotation Matrix  InputEulerSequence=ZYX  ShowTrVecInputPort=on  OutputRepresentation=Euler Angles  OutputEulerSequence=XYZ  ShowTrVecOutputPort=on  SimulateUsing=Interpreted execution
      settings: LibrarySourceBlock=navlib/Utilities/Coordinate Transformation Conversion
  Divide1 : Product  Inputs=*/  Multiplication=Matrix(*)
  Environmental Forces and Moments : AUVLib/Environmental Forces and Moments  V=4.041e-5  h=0.01  mass=0.02  CoB=[0; 0; 0]  Hy=Simple  ang_coeff="diag([ 0.3,  2,  20])"  quad_coeff="diag([ 0.05,  1.5,  1.6])"  lin_coeff="diag([ 0.05,  1.5,  1.5])"  ang_coeff_c="diag([ 10, 80,  82])"  alphaR=0  betaR=0  CX=0  CY=0  CZ=0  CMK=0  CMM=0  CMN=0  inputAxes=Body  cbar=1  b=1  S=1
  Subsystem1 : Subsystem
  Torpedo Pose : Outport
  wires:
  Bus Creator/1 -> Environmental Forces and Moments/1  "tropedo_state"
  Initial_state/1 -> Subsystem1/1(init_state)
  Coordinate Transformation Conversion4/1 -> Bus Creator1/1  "orientation_topedo"
  Bus Creator1/1 -> Torpedo Pose/1
  Environmental Forces and Moments/1 -> 6DOF (Quaternion)/1
  Environmental Forces and Moments/2 -> 6DOF (Quaternion)/2
  6DOF (Quaternion)/2 -> Subsystem1/2(pos_e)  "Position_e"
  6DOF (Quaternion)/5 -> Subsystem1/3(rot_m)  "rotation_matrix"
  6DOF (Quaternion)/7 -> Bus Creator/4  "angular_velocity_b"
  6DOF (Quaternion)/6 -> Bus Creator/3  "Velocity_b"
  Subsystem1/1(Position_e) -> Bus Creator/1, Bus Creator1/2
  Subsystem1/2(rotation_matrix) -> Divide1/2, Bus Creator/2
  Constant1/1 -> Divide1/1
  Divide1/1 -> Coordinate Transformation Conversion4/1  "rotation_matrix"

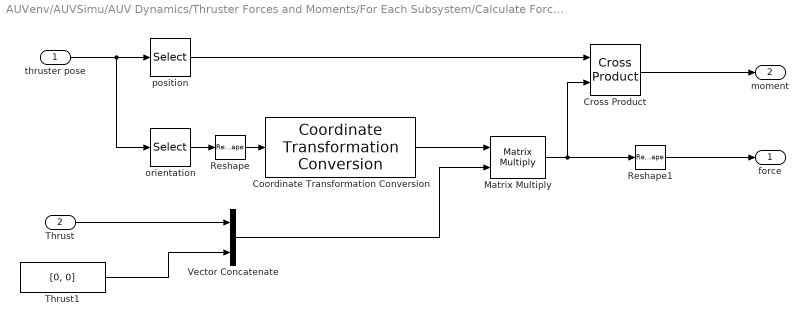
== system AUVenv/AUVSimu/AUV Dynamics/Thruster Forces and Moments/For Each Subsystem/Calculate Force and Moment ==
  thruster pose : Inport
  Thrust : Inport  Port=2
  Coordinate Transformation Conversion : robotcorelib/Coordinate Transformation Conversion  InputRepresentation=Euler Angles  InputEulerSequence=XYZ  ShowTrVecInputPort=on  OutputRepresentation=Rotation Matrix  OutputEulerSequence=ZYX  ShowTrVecOutputPort=on  SimulateUsing=Interpreted execution
  Cross Product : matrix_library/Cross Product
  Matrix Multiply : Product  Multiplication=Matrix(*)
  Reshape : Reshape  OutputDimensionality=Column vector (2-D)
  Reshape1 : Reshape  OutputDimensionality=Row vector (2-D)
  Thrust1 : Constant  Value=[0, 0]
  Vector Concatenate : Concatenate
  orientation : Selector  InputPortWidth=6  IndexOptions=Index vector (dialog)  Indices=[4 5 6]  OutputSizes=1
  position : Selector  InputPortWidth=6  IndexOptions=Index vector (dialog)  Indices=[1 2 3]  OutputSizes=1
  force : Outport
  moment : Outport  Port=2
  wires:
  Vector Concatenate/1 -> Matrix Multiply/2
  Thrust1/1 -> Vector Concatenate/2
  Matrix Multiply/1 -> Reshape1/1, Cross Product/2
  Coordinate Transformation Conversion/1 -> Matrix Multiply/1
  orientation/1 -> Reshape/1
  Thrust/1 -> Vector Concatenate/1
  Cross Product/1 -> moment/1
  thruster pose/1 -> orientation/1, position/1
  position/1 -> Cross Product/1
  Reshape/1 -> Coordinate Transformation Conversion/1
  Reshape1/1 -> force/1

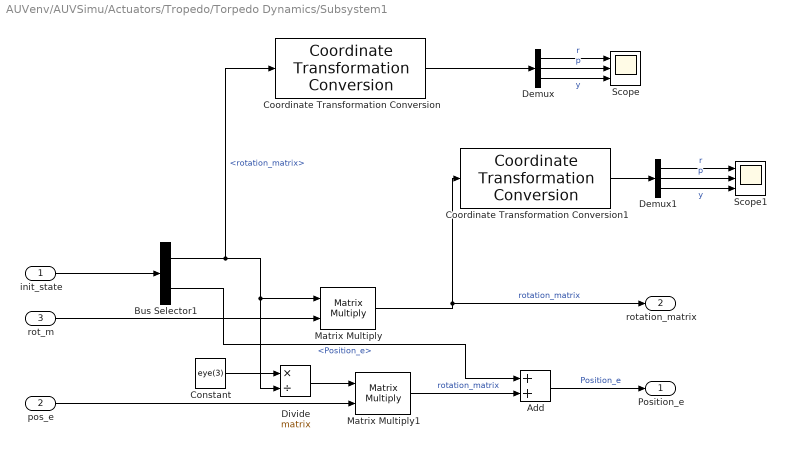
== system AUVenv/AUVSimu/Actuators/Tropedo/Torpedo Dynamics/Subsystem1 ==
  init_state : Inport
  pos_e : Inport  Port=2
  rot_m : Inport  Port=3
  Add : Sum
  Bus Selector1 : BusSelector  OutputSignals=rotation_matrix,Position_e
  Constant : Constant  Value=eye(3)
  Coordinate Transformation Conversion : robotcorelib/Coordinate Transformation Conversion  InputRepresentation=Rotation Matrix  InputEulerSequence=ZYX  ShowTrVecInputPort=on  OutputRepresentation=Euler Angles  OutputEulerSequence=XYZ  ShowTrVecOutputPort=on  SimulateUsing=Interpreted execution
      settings: LibrarySourceBlock=navlib/Utilities/Coordinate Transformation Conversion
  Coordinate Transformation Conversion1 : robotcorelib/Coordinate Transformation Conversion  InputRepresentation=Rotation Matrix  InputEulerSequence=ZYX  ShowTrVecInputPort=on  OutputRepresentation=Euler Angles  OutputEulerSequence=XYZ  ShowTrVecOutputPort=on  SimulateUsing=Interpreted execution
      settings: LibrarySourceBlock=navlib/Utilities/Coordinate Transformation Conversion
  Demux : Demux  Outputs=3
  Demux1 : Demux  Outputs=3
  Divide : Product  Inputs=*/  Multiplication=Matrix(*)
  Matrix Multiply : Product  Multiplication=Matrix(*)
  Matrix Multiply1 : Product  Multiplication=Matrix(*)
  Scope : Scope  NumInputPorts=3
      settings: ActiveDisplayYMinimum=-0.91505450914068209  ActiveDisplayYMaximum=0.11578058031846855  DataLoggingVariableName=ScopeData12
  Scope1 : Scope  NumInputPorts=3
      settings: ActiveDisplayYMinimum=-0.098174770424681021  ActiveDisplayYMaximum=0.88357293382212942  DataLoggingVariableName=ScopeData13
  Position_e : Outport
  rotation_matrix : Outport  Port=2
  wires:
  Bus Selector1/1 -> Coordinate Transformation Conversion/1, Divide/2, Matrix Multiply/1  "<rotation_matrix>"
  Bus Selector1/2 -> Add/1  "<Position_e>"
  init_state/1 -> Bus Selector1/1
  rot_m/1 -> Matrix Multiply/2
  pos_e/1 -> Matrix Multiply1/2
  Constant/1 -> Divide/1
  Divide/1 -> Matrix Multiply1/1
  Matrix Multiply1/1 -> Add/2  "rotation_matrix"
  Add/1 -> Position_e/1  "Position_e"
  Coordinate Transformation Conversion/1 -> Demux/1
  Coordinate Transformation Conversion1/1 -> Demux1/1
  Demux/2 -> Scope/2  "p"
  Demux/1 -> Scope/1  "r"
  Demux/3 -> Scope/3  "y"
  Demux1/1 -> Scope1/1  "r"
  Demux1/2 -> Scope1/2  "p"
  Demux1/3 -> Scope1/3  "y"
  Matrix Multiply/1 -> Coordinate Transformation Conversion1/1, rotation_matrix/1  "rotation_matrix"
